simulink model "B5_simulation_paparazzi"  (R2021b)
settings: Solver=VariableStepAuto  StartTime=0.0  StopTime=5.5  FixedStep=0.002  RelTol=1e-3
values from neighbouring files (symbols this model uses):
  coef_sim_1 = tf_des_d.Denominator{1}(2)    [A11_setup_script_pprz.m]    (also in A1_setup_script.m; A6_slow_actuator.m)
  coef_sim_2 = tf_des_d.Numerator{1}(2)    [A11_setup_script_pprz.m]    (also in A1_setup_script.m; A6_slow_actuator.m)
  coeff = 1    [A11_setup_script_pprz.m]    (also in A12_sim_multi_run.m = coeff_list(i))
  doublet_mag = - 0.15    (= -0.15)    [A11_setup_script_pprz.m]    (also in A1_setup_script.m)
  doublet_time = 6    [A11_setup_script_pprz.m]    (also in A1_setup_script.m)
  f_8 = 1    [A11_setup_script_pprz.m]    (also in A1_setup_script.m)
  FILT_CUTOFF = 2*pi*5    (= 31.4159265359)    [A11_setup_script_pprz.m]    (also in A1_setup_script.m)
  FILTER = 1    [A11_setup_script_pprz.m]    (also in A1_setup_script.m)
  G1 = inv(I)*G1_r    [A10_simple_plant.m]    (also in A11_setup_script_pprz.m = G1/scale; A1_setup_script.m = [G1;G1_T])
  G2 = G2/scale    [A11_setup_script_pprz.m]    (also in A1_setup_script.m = (1/sampling_time)*inv(I)*(G2_r))
  h_plate = 0.3    [A11_setup_script_pprz.m]    (also in A1_setup_script.m = 0.16)
  I = eye(3,3)    [A10_simple_plant.m]    (also in A11_setup_script_pprz.m; A1_setup_script.m; A2_B_matrix_generation_symbolic.m = [Ixx 0 0; A3_B_matrix_generation_symbolic_cascaded.m = [Ixx 0 0)
  Iyy = 0.0008    [A11_setup_script_pprz.m]    (also in A1_setup_script.m = 0.0015)
  K = 7    [A11_setup_script_pprz.m]    (also in A1_setup_script.m = 10)
  K_act = 50    [A10_simple_plant.m]    (also in A11_setup_script_pprz.m = 20; A1_setup_script.m = 20)
  K_d = 15    [A11_setup_script_pprz.m]    (also in A1_setup_script.m = 25)
  K_dd = K_act    (= 20)    [A11_setup_script_pprz.m]    (also in A1_setup_script.m)
  K_ec = 50    [A11_setup_script_pprz.m]    (also in A1_setup_script.m = 251)
  K_ec_d = 13    [A11_setup_script_pprz.m]    (also in A1_setup_script.m = 25)
  K_ec_d_u = 1.5    [A11_setup_script_pprz.m]    (also in A1_setup_script.m = 5)
  K_ec_d_v = 1.5    [A11_setup_script_pprz.m]    (also in A1_setup_script.m = 5)
  K_ec_dd = 9    [A11_setup_script_pprz.m]    (also in A1_setup_script.m = 45)
  K_ec_i = 0    [A11_setup_script_pprz.m]    (also in A1_setup_script.m = 380)
  K_ec_u = 1.5    [A11_setup_script_pprz.m]    (also in A1_setup_script.m = 5)
  K_ec_v = 1.5    [A11_setup_script_pprz.m]    (also in A1_setup_script.m = 5)
  K_t = 0.0005    [A10_simple_plant.m]    (also in A11_setup_script_pprz.m = 6.557e-08; A1_setup_script.m = 6.557e-08)
  K_u = 1.0    (= 1)    [A11_setup_script_pprz.m]    (also in A1_setup_script.m = 1.5)
  K_u_d = 2.5    [A11_setup_script_pprz.m]    (also in A1_setup_script.m = 7)
  K_v = 1.0    (= 1)    [A11_setup_script_pprz.m]    (also in A1_setup_script.m = 1.5)
  K_v_d = 2.5    [A11_setup_script_pprz.m]    (also in A1_setup_script.m = 7)
  K_w = 1.0    (= 1)    [A11_setup_script_pprz.m]    (also in A1_setup_script.m = 4.5)
  K_w_d = 2.5    [A11_setup_script_pprz.m]    (also in A1_setup_script.m = 7)
  l_plate = 0.1    [A11_setup_script_pprz.m]    (also in A1_setup_script.m = 0.11)
  m = 0.4    [A10_simple_plant.m]    (also in A11_setup_script_pprz.m; A1_setup_script.m)
  NOISE = 0    [A11_setup_script_pprz.m]    (also in A1_setup_script.m)
  NOISE_ACC = 0.00005    (= 5e-05)    [A11_setup_script_pprz.m]    (also in A1_setup_script.m)
  NOISE_GYRO = 0.00005    (= 5e-05)    [A11_setup_script_pprz.m]    (also in A1_setup_script.m)
  NOISE_RPM = 200    [A11_setup_script_pprz.m]    (also in A1_setup_script.m)
  omega_des = 20.00    (= 20)    [A11_setup_script_pprz.m]    (also in A1_setup_script.m; A6_slow_actuator.m = 49)
  sampling_time = 1/frequency    (= 0.002)    [A11_setup_script_pprz.m]    (also in A12_sim_multi_run.m; A1_setup_script.m; A6_slow_actuator.m)
  scale_8 = 1.6    [A11_setup_script_pprz.m]    (also in A1_setup_script.m)
  start_8 = 2    [A11_setup_script_pprz.m]    (also in A1_setup_script.m)
  start_time = 2    [A11_setup_script_pprz.m]    (also in A1_setup_script.m = 1)
  t_8 = 10    [A11_setup_script_pprz.m]    (also in A1_setup_script.m)
  w_plate = 0.3    [A11_setup_script_pprz.m]    (also in A1_setup_script.m = 0.36)
undefined symbols (not defined in the file or in its folder): DiscIntNeverNeededParam
libraries: simulink x11, cstblocks x9, dspinverses x8, dspmathops x4, dspstat3 x4, aerolibutil x3, sharedutil x2, aerolibanim x1
(part 5 of 5)

== matlab function B5_simulation_paparazzi/Model Block Complementary Filters/Extended INDI/Subsystem/MATLAB Function ==
  data: theta input; qdd_comp output; dtheta input; Vx input; Vy input; Vz input; Ax input; Ay input; Az input; u input; w_plate input; h_plate input; l_plate input; Iyy input
function qdd_comp = fcn(theta,dtheta,Vx,Vy,Vz,Ax,Ay,Az,u,w_plate,h_plate,l_plate,Iyy)

S_plate = w_plate * h_plate;
rho = 1.225;
Cd1 = 0.0033;
Cd2 = 0.7;
Cl1 = -0.0228;
Cl2 = 2.01;

qdd_comp = - (dtheta*l_plate*sign(u)*((S_plate*rho*cos((pi*((180*theta)/pi + (180*atan2(Vz, (Vx^2 + Vy^2)^(1/2)))/pi))/180)*(Cl2 + Cl1*((180*theta)/pi + (180*atan2(Vz, (Vx^2 + Vy^2)^(1/2)))/pi + 90))*(Vx^2 + Vy^2 + Vz^2))/2 + (S_plate*rho*sin((pi*((180*theta)/pi + (180*atan2(Vz, (Vx^2 + Vy^2)^(1/2)))/pi))/180)*(Cd2 + Cd1*((180*theta)/pi + (180*atan2(Vz, (Vx^2 + Vy^2)^(1/2)))/pi + 90))*(Vx^2 + Vy^2 + Vz^2))/2 - (90*Cd1*S_plate*rho*cos((pi*((180*theta)/pi + (180*atan2(Vz, (Vx^2 + Vy^2)^(1/2)))/pi))/180)*(Vx^2 + Vy^2 + Vz^2))/pi + (90*Cl1*S_plate*rho*sin((pi*((180*theta)/pi + (180*atan2(Vz, (Vx^2 + Vy^2)^(1/2)))/pi))/180)*(Vx^2 + Vy^2 + Vz^2))/pi))/Iyy + (Ax*l_plate*sign(u)*(- S_plate*Vx*rho*sin((pi*((180*theta)/pi + (180*atan2(Vz, (Vx^2 + Vy^2)^(1/2)))/pi))/180)*(Cl2 + Cl1*((180*theta)/pi + (180*atan2(Vz, (Vx^2 + Vy^2)^(1/2)))/pi + 90)) + S_plate*Vx*rho*cos((pi*((180*theta)/pi + (180*atan2(Vz, (Vx^2 + Vy^2)^(1/2)))/pi))/180)*(Cd2 + Cd1*((180*theta)/pi + (180*atan2(Vz, (Vx^2 + Vy^2)^(1/2)))/pi + 90)) + (S_plate*Vx*Vz*rho*cos((pi*((180*theta)/pi + (180*atan2(Vz, (Vx^2 + Vy^2)^(1/2)))/pi))/180)*(Cl2 + Cl1*((180*theta)/pi + (180*atan2(Vz, (Vx^2 + Vy^2)^(1/2)))/pi + 90)))/(2*(Vx^2 + Vy^2)^(1/2)) + (S_plate*Vx*Vz*rho*sin((pi*((180*theta)/pi + (180*atan2(Vz, (Vx^2 + Vy^2)^(1/2)))/pi))/180)*(Cd2 + Cd1*((180*theta)/pi + (180*atan2(Vz, (Vx^2 + Vy^2)^(1/2)))/pi + 90)))/(2*(Vx^2 + Vy^2)^(1/2)) - (90*Cd1*S_plate*Vx*Vz*rho*cos((pi*((180*theta)/pi + (180*atan2(Vz, (Vx^2 + Vy^2)^(1/2)))/pi))/180))/(pi*(Vx^2 + Vy^2)^(1/2)) + (90*Cl1*S_plate*Vx*Vz*rho*sin((pi*((180*theta)/pi + (180*atan2(Vz, (Vx^2 + Vy^2)^(1/2)))/pi))/180))/(pi*(Vx^2 + Vy^2)^(1/2))))/Iyy + (Ay*l_plate*sign(u)*(- S_plate*Vy*rho*sin((pi*((180*theta)/pi + (180*atan2(Vz, (Vx^2 + Vy^2)^(1/2)))/pi))/180)*(Cl2 + Cl1*((180*theta)/pi + (180*atan2(Vz, (Vx^2 + Vy^2)^(1/2)))/pi + 90)) + S_plate*Vy*rho*cos((pi*((180*theta)/pi + (180*atan2(Vz, (Vx^2 + Vy^2)^(1/2)))/pi))/180)*(Cd2 + Cd1*((180*theta)/pi + (180*atan2(Vz, (Vx^2 + Vy^2)^(1/2)))/pi + 90)) + (S_plate*Vy*Vz*rho*cos((pi*((180*theta)/pi + (180*atan2(Vz, (Vx^2 + Vy^2)^(1/2)))/pi))/180)*(Cl2 + Cl1*((180*theta)/pi + (180*atan2(Vz, (Vx^2 + Vy^2)^(1/2)))/pi + 90)))/(2*(Vx^2 + Vy^2)^(1/2)) + (S_plate*Vy*Vz*rho*sin((pi*((180*theta)/pi + (180*atan2(Vz, (Vx^2 + Vy^2)^(1/2)))/pi))/180)*(Cd2 + Cd1*((180*theta)/pi + (180*atan2(Vz, (Vx^2 + Vy^2)^(1/2)))/pi + 90)))/(2*(Vx^2 + Vy^2)^(1/2)) - (90*Cd1*S_plate*Vy*Vz*rho*cos((pi*((180*theta)/pi + (180*atan2(Vz, (Vx^2 + Vy^2)^(1/2)))/pi))/180))/(pi*(Vx^2 + Vy^2)^(1/2)) + (90*Cl1*S_plate*Vy*Vz*rho*sin((pi*((180*theta)/pi + (180*atan2(Vz, (Vx^2 + Vy^2)^(1/2)))/pi))/180))/(pi*(Vx^2 + Vy^2)^(1/2))))/Iyy - (Az*l_plate*sign(u)*(S_plate*Vz*rho*sin((pi*((180*theta)/pi + (180*atan2(Vz, (Vx^2 + Vy^2)^(1/2)))/pi))/180)*(Cl2 + Cl1*((180*theta)/pi + (180*atan2(Vz, (Vx^2 + Vy^2)^(1/2)))/pi + 90)) + (S_plate*rho*cos((pi*((180*theta)/pi + (180*atan2(Vz, (Vx^2 + Vy^2)^(1/2)))/pi))/180)*(Vx^2 + Vy^2)^(1/2)*(Cl2 + Cl1*((180*theta)/pi + (180*atan2(Vz, (Vx^2 + Vy^2)^(1/2)))/pi + 90)))/2 + (S_plate*rho*sin((pi*((180*theta)/pi + (180*atan2(Vz, (Vx^2 + Vy^2)^(1/2)))/pi))/180)*(Vx^2 + Vy^2)^(1/2)*(Cd2 + Cd1*((180*theta)/pi + (180*atan2(Vz, (Vx^2 + Vy^2)^(1/2)))/pi + 90)))/2 - S_plate*Vz*rho*cos((pi*((180*theta)/pi + (180*atan2(Vz, (Vx^2 + Vy^2)^(1/2)))/pi))/180)*(Cd2 + Cd1*((180*theta)/pi + (180*atan2(Vz, (Vx^2 + Vy^2)^(1/2)))/pi + 90)) - (90*Cd1*S_plate*rho*cos((pi*((180*theta)/pi + (180*atan2(Vz, (Vx^2 + Vy^2)^(1/2)))/pi))/180)*(Vx^2 + Vy^2)^(1/2))/pi + (90*Cl1*S_plate*rho*sin((pi*((180*theta)/pi + (180*atan2(Vz, (Vx^2 + Vy^2)^(1/2)))/pi))/180)*(Vx^2 + Vy^2)^(1/2))/pi))/Iyy;

== matlab function B5_simulation_paparazzi/Model Block Complementary Filters/Force and Moment Calculation/Drag Plate Aerodynamics/drag plate My1 ==
  data: w_plate input; h_plate input; l_plate input; theta input; Vx input; Cd output; Cl output; Vx output; Vy output; Vy input; Vz input; Vz output; gamma output; theta output; alpha output; D_plate output; L_plate output; R_plate output; u input; My_dp output
function [Cd,Cl,Vx,Vy,Vz,gamma,theta,alpha,D_plate,L_plate,R_plate,My_dp] = drag_plate_My(w_plate,h_plate,l_plate,theta,Vx,Vy,Vz,u)

% define constants
rho = 1.225;
S_plate = w_plate*h_plate;

% Resultant
Vr = sqrt(Vx^2+Vy^2+Vz^2);
Vh = sqrt(Vx^2+Vy^2);

gamma = -rad2deg(atan2(Vz,Vh));
theta = rad2deg(theta);

alpha = theta-gamma;

% Drag Coefficient
Cd = 0.0033*(90+alpha)+0.7;

% Lift Coefficient
Cl = -0.0228*(90+alpha)+2.01;

% get drag and lift
D_plate= 0.5*rho*Vr^2*S_plate*Cd;
L_plate = 0.5*rho*Vr^2*S_plate*Cl;
R_plate = cos(deg2rad(alpha))*D_plate - sin(deg2rad(alpha))*L_plate;

My_dp = l_plate*R_plate*sign(u);
